simulink model "GSK_PVModel_05"  (R2017a)
settings: Solver=VariableStepAuto  StartTime=0.0  StopTime=10.0  FixedStep=0.001  RelTol=1e-3
values from neighbouring files (symbols this model uses):
  G_n = 1000    [GSK_PVModelValues.m]    (also in GSK_PVModelValues_05.m)
  I_pv_n = 6.5    [GSK_PVModelValues.m]    (also in GSK_PVModelValues_05.m)
  K_I = 3.5e-3    (= 0.0035)    [GSK_PVModelValues.m]    (also in GSK_PVModelValues_05.m)
  T = 273+40    (= 313)    [GSK_PVModelValues.m]    (also in GSK_PVModelValues_05.m)
  T_n = 25+273    (= 298)    [GSK_PVModelValues.m]    (also in GSK_PVModelValues_05.m)
libraries: fl_lib x11, nesl_utility x5, simulink x2, elec_lib x1
settings Model: Creator=gadis  LastModifiedBy=gadis

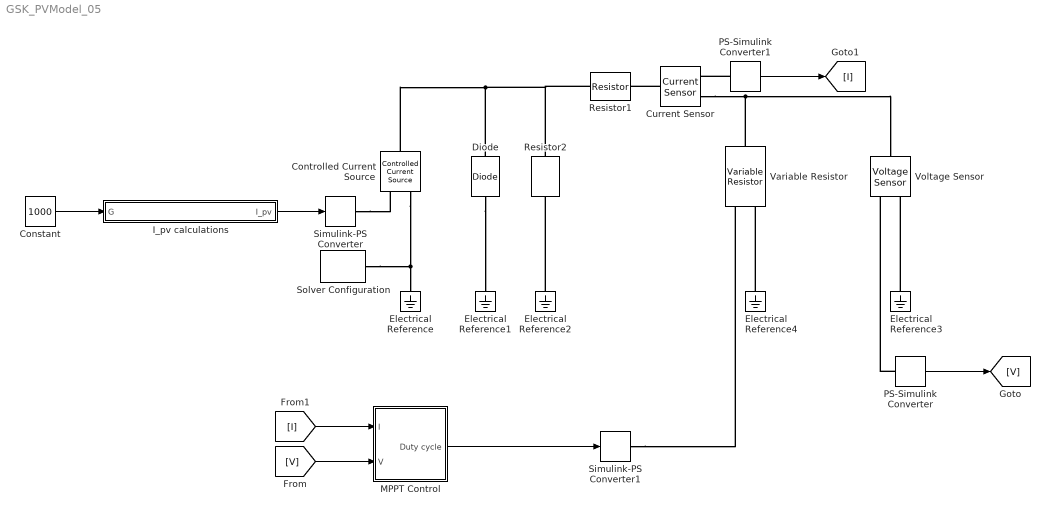
== system GSK_PVModel_05 ==
  Constant : Constant  Value=1000
  Controlled Current Source : fl_lib/Electrical/Electrical Sources/Controlled Current Source
  Current Sensor : fl_lib/Electrical/Electrical Sensors/Current Sensor
  Diode : elec_lib/Semiconductor Devices/Diode  ModelType=3  Vf=0.6 V  Ron=0.3 Ohm  Goff=1e-8 S  Rz=0.3 Ohm  Vz=50 V  C_PWL=5 pF  prmExp=1  I12=[ 3.9574e-05 0.0914 ] A  V12=[ 20 60 ] V  I1=0.0137 A  V1=0.6 V  IS=1e-12 A  ec=1  RS=0.01 Ohm  Tmeas=25 degC  BV=Inf V  C_param=1  CJ0=5 pF  VJ=1 V  Mgrad=0.5  Vvec=[ 0.1 10 100 ] V  Cvec=[ 3.5 1 0.4 ] pF  FC=0.5  Q_param=1  Irrm=-7.15 A  iF=4 A  didt=-750 A/us  trr=115 ns  TT=50 ns  tau=100 ns  T_param=1  IS_T2=1.25e-7 A  I1_T2=0.245 A  V1_T2=0.5 V  Tmeas2=125 degC  EG_param=1  EG=1.11 eV  XTI_param=1  XTI=3  dBVdT=0 V/K  Tdevice=25 degC  i_capacitor_specify=off  i_capacitor_priority=High  i_capacitor=0 A  i_capacitor_nominal_specify=off  i_capacitor_nominal_unit=A  i_capacitor_nominal_value=1  v_capacitor_specify=off  v_capacitor_priority=None  v_capacitor=0 V  v_capacitor_nominal_specify=off  v_capacitor_nominal_unit=V  v_capacitor_nominal_value=1  Rth=[ 0 10 ] K/W  thermal_mass_parameterization=1  thermal_mass=[ 0 1 ] J/K  thermal_time_constant=[ 0 10 ] s  thermal_mass_initial_temperatures=[ 25 25 ] degC
      settings: SourceProductName=Simscape Electronics  SourceProductBaseCode=SN
  Electrical Reference{,1..4} (5 alike) : fl_lib/Electrical/Electrical Elements/Electrical Reference
  I_pv calculations : Subsystem
  MPPT Control : Subsystem
  PS-Simulink Converter : nesl_utility/PS-Simulink Converter  PhysicalDomain=network_engine_domain  SubClassName=ps_output  LeftPortType=input  RightPortType=output  PseudoPeriodic=off  Frequencies=[]  Unit=1  AffineConversion=off
  PS-Simulink Converter1 : nesl_utility/PS-Simulink Converter  PhysicalDomain=network_engine_domain  SubClassName=ps_output  LeftPortType=input  RightPortType=output  PseudoPeriodic=off  Frequencies=[]  Unit=1  AffineConversion=off
  Resistor1 : fl_lib/Electrical/Electrical Elements/Resistor  R=1e-3*128 Ohm  i_specify=off  i_priority=None  i=0 A  i_nominal_specify=off  i_nominal_unit=A  i_nominal_value=1  v_specify=off  v_priority=None  v=0 V  v_nominal_specify=off  v_nominal_unit=V  v_nominal_value=1
  Resistor2 : fl_lib/Electrical/Electrical Elements/Resistor  R=1000 Ohm  i_specify=off  i_priority=None  i=0 A  i_nominal_specify=off  i_nominal_unit=A  i_nominal_value=1  v_specify=off  v_priority=None  v=0 V  v_nominal_specify=off  v_nominal_unit=V  v_nominal_value=1
  Simulink-PS Converter : nesl_utility/Simulink-PS Converter  PhysicalDomain=network_engine_domain  SubClassName=ps_input  LeftPortType=input  RightPortType=output  PseudoPeriodic=off  Frequencies=[]  NoiseDistribution=none  NoiseParameters=[]  Unit=1  AffineConversion=off  FilteringAndDerivatives=zero  SimscapeFilterOrder=1  InputFilterTimeConstant=0.001  UdotUserProvided=1
  Simulink-PS Converter1 : nesl_utility/Simulink-PS Converter  PhysicalDomain=network_engine_domain  SubClassName=ps_input  LeftPortType=input  RightPortType=output  PseudoPeriodic=off  Frequencies=[]  NoiseDistribution=none  NoiseParameters=[]  Unit=1  AffineConversion=off  FilteringAndDerivatives=zero  SimscapeFilterOrder=1  InputFilterTimeConstant=0.001  UdotUserProvided=1
  Solver Configuration : nesl_utility/Solver Configuration  PhysicalDomain=network_engine_domain  SubClassName=solver  LeftPortType=input  RightPortType=generic  Accelerate=off  Tones=[]  Harmonics=[]  SimulateNoise=off  Profile=off  UseLocalSampling=off  EnableSwitchedLinearOptims=on  FrequencyDomain=off  UseCCode=off  RelTol=0.001  AbsTol=1e-06  MinStep=1e-09  ToWorkspace=off  RevertToSquareIcSolve=off  NumHomotopyIterations=100  PhasorMode=off  PhasorModeNumHarmonics=1  OverrideAbsTol=off  DoDC=on  ResidualTolerance=1e-09  UseLocalSolver=off  LocalSolverChoice=NE_BACKWARD_EULER_ADVANCER  LocalSolverSampleTime=0.001  DoFixedCost=off  MaxNonlinIter=3  MaxModeIter=2  LinearAlgebra=Sparse  DelaysMemoryBudget=1024  AutomaticFiltering=on  FilteringTimeConstant=0.001
  Variable Resistor : fl_lib/Electrical/Electrical Elements/Variable Resistor  Rmin=0.01 Ohm  i_specify=off  i_priority=None  i=0 A  i_nominal_specify=off  i_nominal_unit=A  i_nominal_value=1  v_specify=off  v_priority=None  v=0 V  v_nominal_specify=off  v_nominal_unit=V  v_nominal_value=1
  Voltage Sensor : fl_lib/Electrical/Electrical Sensors/Voltage Sensor
  wires:
  I_pv calculations/1(I_pv) -> Simulink-PS Converter/1
  Constant/1 -> I_pv calculations/1(G)
  MPPT Control/1(Duty cycle) -> Simulink-PS Converter1/1
  PS-Simulink Converter/1 -> [V]
  [V] -> MPPT Control/2(V)
  PS-Simulink Converter1/1 -> [I]
  [I] -> MPPT Control/1(I)
  connections:
  Controlled Current Source/RConn2 -- Solver Configuration/RConn1 -- Electrical Reference/LConn1
  Simulink-PS Converter/RConn1 -- Controlled Current Source/RConn1
  Controlled Current Source/LConn1 -- Diode/LConn1 -- Resistor1/LConn1 -- Resistor2/LConn1
  Diode/RConn1 -- Electrical Reference1/LConn1
  Electrical Reference2/LConn1 -- Resistor2/RConn1
  Electrical Reference4/LConn1 -- Variable Resistor/LConn2
  Simulink-PS Converter1/RConn1 -- Variable Resistor/LConn1
  Variable Resistor/RConn1 -- Current Sensor/RConn2 -- Voltage Sensor/LConn1
  Electrical Reference3/LConn1 -- Voltage Sensor/RConn2
  PS-Simulink Converter/LConn1 -- Voltage Sensor/RConn1
  Current Sensor/LConn1 -- Resistor1/RConn1
  PS-Simulink Converter1/LConn1 -- Current Sensor/RConn1

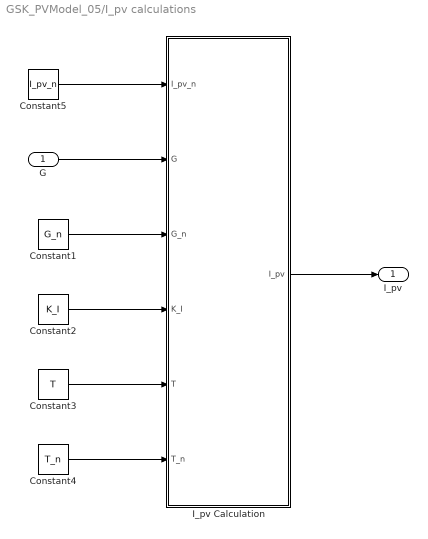
== system GSK_PVModel_05/I_pv calculations ==
  G : Inport
  Constant1 : Constant  Value=G_n
  Constant2 : Constant  Value=K_I
  Constant3 : Constant  Value=T
  Constant4 : Constant  Value=T_n
  Constant5 : Constant  Value=I_pv_n
  I_pv Calculation : MATLAB Function  TreatAsAtomicUnit=on
  I_pv : Outport
  wires:
  Constant5/1 -> I_pv Calculation/1(I_pv_n)
  G/1 -> I_pv Calculation/2(G)
  I_pv Calculation/1(I_pv) -> I_pv/1
  Constant1/1 -> I_pv Calculation/3(G_n)
  Constant2/1 -> I_pv Calculation/4(K_I)
  Constant3/1 -> I_pv Calculation/5(T)
  Constant4/1 -> I_pv Calculation/6(T_n)

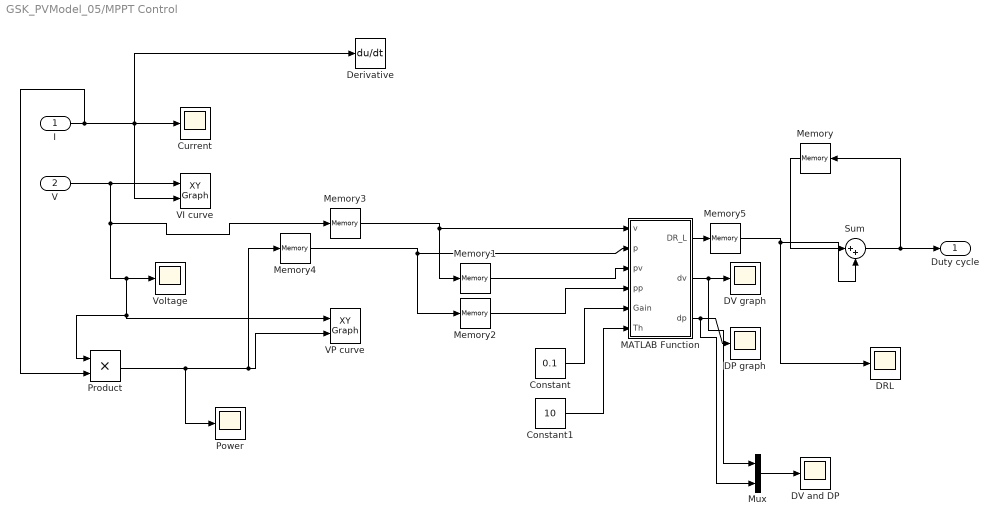
== system GSK_PVModel_05/MPPT Control ==
  I : Inport
  V : Inport  Port=2
  Constant : Constant  Value=0.1
  Constant1 : Constant  Value=10
  Current : Scope
  DP graph : Scope
  DRL : Scope
  DV and DP : Scope
  DV graph : Scope
  Derivative : Derivative
  MATLAB Function : MATLAB Function  TreatAsAtomicUnit=on
  Memory : Memory  X0=2
  Memory{1..5} (5 alike) : Memory
  Mux : Mux  Inputs=2
  Power : Scope
  Product : Product
  Sum : Sum  Inputs=|++
  VI curve : simulink/Sinks/XY Graph  xmin=0  xmax=100  ymin=0  ymax=10  st=-1
  VP curve : simulink/Sinks/XY Graph  xmin=0  xmax=100  ymin=0  ymax=500  st=-1
  Voltage : Scope
  Duty cycle : Outport
  wires:
  V/1 -> VI curve/1, Memory3/1, VP curve/1, Product/1, Voltage/1
  I/1 -> VI curve/2, Derivative/1, Current/1, Product/2
  Product/1 -> Power/1, Memory4/1, VP curve/2
  Constant/1 -> MATLAB Function/5(Gain)
  MATLAB Function/1(DR_L) -> Memory5/1
  Sum/1 -> Memory/1, Duty cycle/1
  Memory/1 -> Sum/1
  Memory1/1 -> MATLAB Function/3(pv)
  Memory2/1 -> MATLAB Function/4(pp)
  Memory3/1 -> MATLAB Function/1(v), Memory1/1
  MATLAB Function/2(dv) -> Mux/1, DV graph/1
  MATLAB Function/3(dp) -> Mux/2, DP graph/1
  Memory4/1 -> Memory2/1, MATLAB Function/2(p)
  Mux/1 -> DV and DP/1
  Constant1/1 -> MATLAB Function/6(Th)
  Memory5/1 -> DRL/1, Sum/2

== matlab function GSK_PVModel_05/I_pv calculations/I_pv Calculation ==
  data: I_pv_n input; I_pv output; G input; G_n input; K_I input; T input; T_n input
function I_pv = fcn(I_pv_n, G, G_n, K_I, T, T_n )
%#codegen
Delta_T = (T - T_n);
I_pv = (I_pv_n + K_I*Delta_T)*G/G_n;

== matlab function GSK_PVModel_05/MPPT Control/MATLAB Function ==
  data: v input; p input; pv input; pp input; DR_L output; Gain input; dv output; dp output; Th input
function [DR_L, dv, dp] = fcn(v, p, pv, pp, Gain, Th)
dv = v - pv;
dp = p - pp;
DR_L = 0;
if (dv == 0)
    DR_L = Gain;
    return
end
if ((dv > 0 && dp > 0) || (dv < 0 && dp < 0) )
    if (dp/dv>=Th)
        DR_L = +Gain;
    else
        DR_L = +0;
    end
    return
 elseif ((dv < 0 && dp > 0) || (dv > 0 && dp < 0) )
     DR_L = -Gain;
     return
end
